simulink model "MLC_LQG_Sim"  (R2019b)
settings: Solver=VariableStepAuto  StartTime=0.0  StopTime=20.0  RelTol=1e-3
values from neighbouring files (symbols this model uses):
  KF_sys = ss(A,B,C,D)    [MLC_LQG.m]
  Q_cost = [1 0; 0 1]    [MLC_LQG.m]
  R_cost = 1    [MLC_LQG.m]
undefined symbols (not defined in the file or in its folder): m_coeff
settings Model: Creator=idelafuentef  LastModifiedBy=idelafuentef

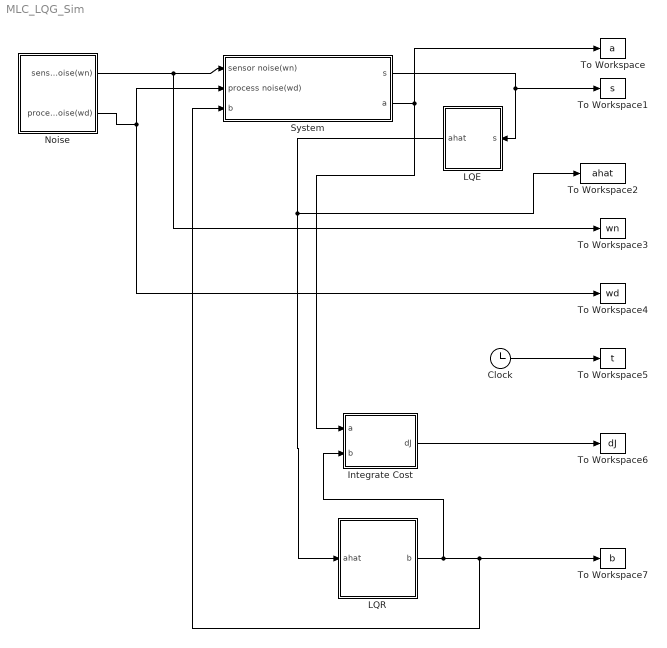
== system MLC_LQG_Sim ==
  Clock : Clock
      settings: Decimation=20
  Integrate Cost : Subsystem
  LQE : Subsystem
  LQR : Subsystem
  Noise : Subsystem
  System : Subsystem
  To Workspace : ToWorkspace  VariableName=a  SaveFormat=Timeseries  SampleTime=-1
  To Workspace1 : ToWorkspace  VariableName=s  SaveFormat=Timeseries  SampleTime=-1
  To Workspace2 : ToWorkspace  VariableName=ahat  SaveFormat=Timeseries  SampleTime=-1
  To Workspace3 : ToWorkspace  VariableName=wn  SaveFormat=Timeseries  SampleTime=-1
  To Workspace4 : ToWorkspace  VariableName=wd  SaveFormat=Timeseries  SampleTime=-1
  To Workspace5 : ToWorkspace  VariableName=t  SaveFormat=Timeseries  SampleTime=-1
  To Workspace6 : ToWorkspace  VariableName=dJ  SaveFormat=Timeseries  SampleTime=-1
  To Workspace7 : ToWorkspace  VariableName=b  SaveFormat=Timeseries  SampleTime=-1
  wires:
  Integrate Cost/1(dJ) -> To Workspace6/1
  LQE/1(ahat) -> To Workspace2/1, LQR/1(ahat)
  Noise/1(sensor noise(wn)) -> To Workspace3/1, System/1(sensor noise(wn))
  Noise/2(process noise(wd)) -> To Workspace4/1, System/2(process noise(wd))
  Clock/1 -> To Workspace5/1
  System/1(s) -> To Workspace1/1, LQE/1(s)
  System/2(a) -> Integrate Cost/1(a), To Workspace/1
  LQR/1(b) -> Integrate Cost/2(b), To Workspace7/1, System/3(b)

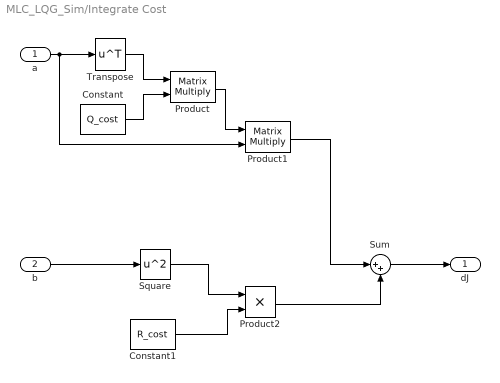
== system MLC_LQG_Sim/Integrate Cost ==
  a : Inport
  b : Inport  Port=2
  Constant : Constant  Value=Q_cost
  Constant1 : Constant  Value=R_cost
  Product : Product  Multiplication=Matrix(*)
  Product1 : Product  Multiplication=Matrix(*)
  Product2 : Product
  Square : Math  Operator=square  SignedPower=off  SaturateOnIntegerOverflow=on
  Sum : Sum  Inputs=|++
  Transpose : Math  Operator=transpose  SignedPower=off  SaturateOnIntegerOverflow=on
  dJ : Outport
  wires:
  Sum/1 -> dJ/1
  a/1 -> Product1/2, Transpose/1
  Transpose/1 -> Product/1
  Constant/1 -> Product/2
  Product/1 -> Product1/1
  Product1/1 -> Sum/1
  b/1 -> Square/1
  Square/1 -> Product2/1
  Constant1/1 -> Product2/2
  Product2/1 -> Sum/2

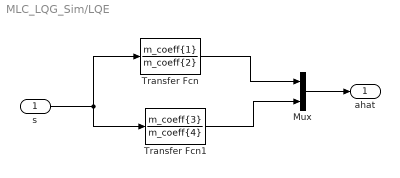
== system MLC_LQG_Sim/LQE ==
  s : Inport
  Mux : Mux  Inputs=2
  Transfer Fcn : TransferFcn  Numerator=m_coeff{1}  Denominator=m_coeff{2}
  Transfer Fcn1 : TransferFcn  Numerator=m_coeff{3}  Denominator=m_coeff{4}
  ahat : Outport
  wires:
  s/1 -> Transfer Fcn1/1, Transfer Fcn/1
  Transfer Fcn/1 -> Mux/1
  Mux/1 -> ahat/1
  Transfer Fcn1/1 -> Mux/2

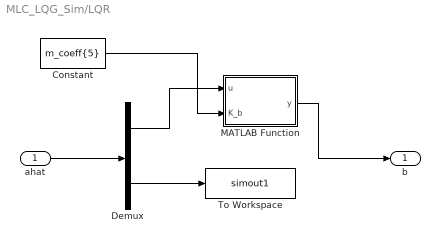
== system MLC_LQG_Sim/LQR ==
  ahat : Inport
  Constant : Constant  Value=m_coeff{5}
  Demux : Demux  Outputs=2
  MATLAB Function : MATLAB Function  TreatAsAtomicUnit=on
  To Workspace : ToWorkspace  VariableName=simout1  SaveFormat=Timeseries  SampleTime=-1
  b : Outport
  wires:
  ahat/1 -> Demux/1
  Demux/1 -> MATLAB Function/1(u)
  MATLAB Function/1(y) -> b/1
  Demux/2 -> To Workspace/1
  Constant/1 -> MATLAB Function/2(K_b)

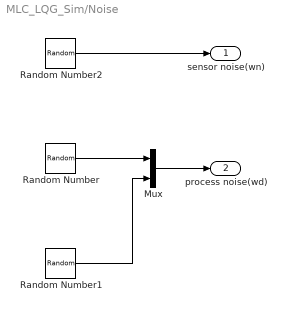
== system MLC_LQG_Sim/Noise ==
  Mux : Mux  Inputs=2
  Random Number : RandomNumber  SampleTime=0.01
  Random Number1 : RandomNumber  Mean=1  SampleTime=0.01
  Random Number2 : RandomNumber  Variance=0.1  SampleTime=0.01
  sensor noise(wn) : Outport
  process noise(wd) : Outport  Port=2  PortDimensions=2
  wires:
  Random Number2/1 -> sensor noise(wn)/1
  Random Number/1 -> Mux/1
  Random Number1/1 -> Mux/2
  Mux/1 -> process noise(wd)/1

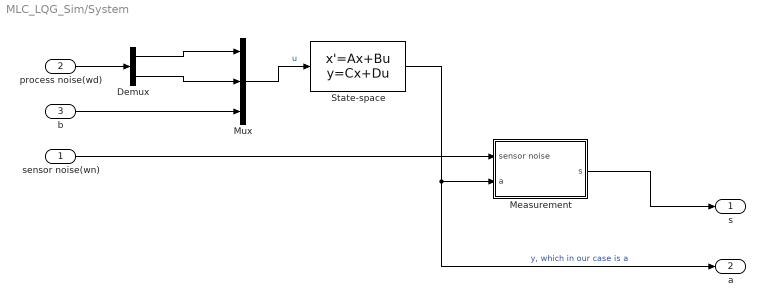
== system MLC_LQG_Sim/System ==
  sensor noise(wn) : Inport
  process noise(wd) : Inport  Port=2
  b : Inport  Port=3
  Demux : Demux  Outputs=2
  Measurement : Subsystem
  Mux : Mux  Inputs=3
  State-space : StateSpace  A=KF_sys.A  B=KF_sys.B  C=KF_sys.C  D=KF_sys.D  InitialCondition=[1 0]
  s : Outport
  a : Outport  Port=2
  wires:
  State-space/1 -> Measurement/2(a), a/1  "y, which in our case is a"
  Measurement/1(s) -> s/1
  sensor noise(wn)/1 -> Measurement/1(sensor noise)
  process noise(wd)/1 -> Demux/1
  Demux/1 -> Mux/1
  Mux/1 -> State-space/1  "u"
  Demux/2 -> Mux/2
  b/1 -> Mux/3

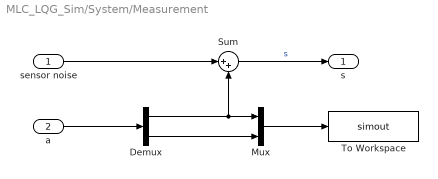
== system MLC_LQG_Sim/System/Measurement ==
  sensor noise : Inport
  a : Inport  Port=2
  Demux : Demux  Outputs=2
  Mux : Mux  Inputs=2
  Sum : Sum  Inputs=|++
  To Workspace : ToWorkspace  VariableName=simout  SaveFormat=Timeseries  SampleTime=-1
  s : Outport
  wires:
  Sum/1 -> s/1  "s"
  Demux/1 -> Mux/1, Sum/2
  sensor noise/1 -> Sum/1
  a/1 -> Demux/1
  Demux/2 -> Mux/2
  Mux/1 -> To Workspace/1

== matlab function MLC_LQG_Sim/LQR/MATLAB Function ==
  data: u input; y output; K_b input
function y = fcn(u,K_b)
    y=0;
    for i=1:length(K_b)
        y=y+K_b(i)*u^(i-1);
    end
end
